simulink model "irep_single_axis"  (Simulink 7.5)
settings: Solver=ode3  StartTime=0.0  StopTime=inf  FixedStep=dt  RelTol=1e-3
InitFcn:
  | IREPOLD_DEPENDENCY
  | init_omni
  | init_filters
  | init_invivo
  | init_telemanipulation
  | init_parker_xyz
  | init_magnetic_tracker
  | init_loadcell
  | init_scopes
  | init_homing
  | init_force_control
  | ATI_Init_nano17
undefined symbols (not defined in the file): A, ATI_torque_convert_to_Nmm, counter_offset, DiscIntNeverNeededParam, dt, encoder_counts, filter_coeffs_ATI, filter_coeffs_ATI_bias, gear_ratio, HomingFineEps, HomingRoughEps, HomingRoughVelocity, inv_T, joystick_filter_coeffs, K_d, K_i, K_p, left_arm_home_voltage, N_ATI, N_ATI_bias, N_joystick, N_pots, pots_filter_coeffs, quadrature_mode, right_arm_home_voltage, RightArmHomingDirectionVector, RightArmHomingIntGain, screw_pitch
libraries: xpcconteclib x23, xpcmeasurementcomputinglib x17, xpclib x11, simulink x8, dspswit3 x4, dspsigops x1, powerlib_extras x1
(part 2 of 3)

== system irep_single_axis/In-Vivo System/CONTEC CARDS/Level 3 ==
  Mux : Mux  Inputs=5
  camera: open joint : xpcconteclib/Incremental Encoder/CNT32-8M(PCI)   Channel=5  OperationMode=2-phase Input Synchronous Clear Multiply by 4  DigitalFilter=No filtering  PulseInput=TTL level input  Direction=Up in the clockwise direction/Down in the counterclockwise direction  InitialValue=counter_offset_init  LoadInitialValue=on  SampleTime=dt  PciSlot=[2,11]  StartMethod=Model Start  StopMethod=Model Terminate  ZeroClearRising=off  ZeroClearFalling=off  ZeroClearMatch0=off  ZeroClearMatch1=off  PresetRising=off  PresetFalling=off  PresetMatch0=off  PresetMatch1=off  PresetValue=0  Match0Value=0  Match1Value=0  OutputSignalMatch0=off  OutputSignalMatch1=off  OutputSignalAbnormal=off  OutputSignalDigitalFilter=off  OutputSignalAlarm=off  OneShotDuration=10 microseconds  IndexEnable=Disable  IndexLogic=Positive (Active High)  EnableDigitalInput=off  EnableDigitalOutput=off  DigitalOutputInitialValue=None  DigitalOutputFinalValue=None
  camera: open joint1 : xpcconteclib/Incremental Encoder/CNT32-8M(PCI)   Channel=6  OperationMode=2-phase Input Synchronous Clear Multiply by 4  DigitalFilter=No filtering  PulseInput=TTL level input  Direction=Up in the clockwise direction/Down in the counterclockwise direction  InitialValue=counter_offset_init  LoadInitialValue=on  SampleTime=dt  PciSlot=[2,11]  StartMethod=Model Start  StopMethod=Model Terminate  ZeroClearRising=off  ZeroClearFalling=off  ZeroClearMatch0=off  ZeroClearMatch1=off  PresetRising=off  PresetFalling=off  PresetMatch0=off  PresetMatch1=off  PresetValue=0  Match0Value=0  Match1Value=0  OutputSignalMatch0=off  OutputSignalMatch1=off  OutputSignalAbnormal=off  OutputSignalDigitalFilter=off  OutputSignalAlarm=off  OneShotDuration=10 microseconds  IndexEnable=Disable  IndexLogic=Positive (Active High)  EnableDigitalInput=off  EnableDigitalOutput=off  DigitalOutputInitialValue=None  DigitalOutputFinalValue=None
  camera: open joint2 : xpcconteclib/Incremental Encoder/CNT32-8M(PCI)   Channel=7  OperationMode=2-phase Input Synchronous Clear Multiply by 4  DigitalFilter=No filtering  PulseInput=TTL level input  Direction=Up in the clockwise direction/Down in the counterclockwise direction  InitialValue=counter_offset_init  LoadInitialValue=on  SampleTime=dt  PciSlot=[2,11]  StartMethod=Model Start  StopMethod=Model Terminate  ZeroClearRising=off  ZeroClearFalling=off  ZeroClearMatch0=off  ZeroClearMatch1=off  PresetRising=off  PresetFalling=off  PresetMatch0=off  PresetMatch1=off  PresetValue=0  Match0Value=0  Match1Value=0  OutputSignalMatch0=off  OutputSignalMatch1=off  OutputSignalAbnormal=off  OutputSignalDigitalFilter=off  OutputSignalAlarm=off  OneShotDuration=10 microseconds  IndexEnable=Disable  IndexLogic=Positive (Active High)  EnableDigitalInput=off  EnableDigitalOutput=off  DigitalOutputInitialValue=None  DigitalOutputFinalValue=None
  left arm: insertion : xpcconteclib/Incremental Encoder/CNT32-8M(PCI)   Channel=4  OperationMode=2-phase Input Synchronous Clear Multiply by 4  DigitalFilter=No filtering  PulseInput=TTL level input  Direction=Up in the clockwise direction/Down in the counterclockwise direction  InitialValue=counter_offset_init  LoadInitialValue=on  SampleTime=dt  PciSlot=[2,11]  StartMethod=Model Start  StopMethod=Model Terminate  ZeroClearRising=off  ZeroClearFalling=off  ZeroClearMatch0=off  ZeroClearMatch1=off  PresetRising=off  PresetFalling=off  PresetMatch0=off  PresetMatch1=off  PresetValue=0  Match0Value=0  Match1Value=0  OutputSignalMatch0=off  OutputSignalMatch1=off  OutputSignalAbnormal=off  OutputSignalDigitalFilter=off  OutputSignalAlarm=off  OneShotDuration=10 microseconds  IndexEnable=Disable  IndexLogic=Positive (Active High)  EnableDigitalInput=off  EnableDigitalOutput=off  DigitalOutputInitialValue=None  DigitalOutputFinalValue=None
  right arm: insertion : xpcconteclib/Incremental Encoder/CNT32-8M(PCI)   Channel=1  OperationMode=2-phase Input Synchronous Clear Multiply by 4  DigitalFilter=No filtering  PulseInput=TTL level input  Direction=Up in the clockwise direction/Down in the counterclockwise direction  InitialValue=counter_offset_init  LoadInitialValue=on  SampleTime=dt  PciSlot=[2,11]  StartMethod=Model Start  StopMethod=Model Terminate  ZeroClearRising=off  ZeroClearFalling=off  ZeroClearMatch0=off  ZeroClearMatch1=off  PresetRising=on  PresetFalling=off  PresetMatch0=off  PresetMatch1=off  PresetValue=0  Match0Value=0  Match1Value=0  OutputSignalMatch0=off  OutputSignalMatch1=off  OutputSignalAbnormal=off  OutputSignalDigitalFilter=off  OutputSignalAlarm=off  OneShotDuration=10 microseconds  IndexEnable=Disable  IndexLogic=Positive (Active High)  EnableDigitalInput=off  EnableDigitalOutput=off  DigitalOutputInitialValue=None  DigitalOutputFinalValue=None
  Out1 : Outport
  wires:
  Mux/1 -> Out1/1
  left arm: insertion/1 -> Mux/2
  right arm: insertion/1 -> Mux/1
  camera: open joint/1 -> Mux/3
  camera: open joint1/1 -> Mux/4
  camera: open joint2/1 -> Mux/5

== system irep_single_axis/In-Vivo System/CONTEC CARDS/RZ ==
  CNT32-8M(PCI) Ch1 : xpcconteclib/Incremental Encoder/CNT32-8M(PCI)   Channel=1  OperationMode=2-phase Input Synchronous Clear Multiply by 4  DigitalFilter=No filtering  PulseInput=Differential line receiver input  Direction=Up in the clockwise direction/Down in the counterclockwise direction  InitialValue=counter_offset  LoadInitialValue=on  SampleTime=dt  PciSlot=[2 14]  StartMethod=Model Start  StopMethod=Model Terminate  ZeroClearRising=off  ZeroClearFalling=off  ZeroClearMatch0=off  ZeroClearMatch1=off  PresetRising=off  PresetFalling=off  PresetMatch0=off  PresetMatch1=off  PresetValue=0  Match0Value=0  Match1Value=0  OutputSignalMatch0=off  OutputSignalMatch1=off  OutputSignalAbnormal=off  OutputSignalDigitalFilter=off  OutputSignalAlarm=off  OneShotDuration=10 microseconds  IndexEnable=Disable  IndexLogic=Positive (Active High)  EnableDigitalInput=off  EnableDigitalOutput=off  DigitalOutputInitialValue=None  DigitalOutputFinalValue=None
  CNT32-8M(PCI) Ch2 : xpcconteclib/Incremental Encoder/CNT32-8M(PCI)   Channel=2  OperationMode=2-phase Input Synchronous Clear Multiply by 4  DigitalFilter=No filtering  PulseInput=Differential line receiver input  Direction=Up in the clockwise direction/Down in the counterclockwise direction  InitialValue=counter_offset  LoadInitialValue=on  SampleTime=dt  PciSlot=[2 14]  StartMethod=Model Start  StopMethod=Model Terminate  ZeroClearRising=off  ZeroClearFalling=off  ZeroClearMatch0=off  ZeroClearMatch1=off  PresetRising=off  PresetFalling=off  PresetMatch0=off  PresetMatch1=off  PresetValue=0  Match0Value=0  Match1Value=0  OutputSignalMatch0=off  OutputSignalMatch1=off  OutputSignalAbnormal=off  OutputSignalDigitalFilter=off  OutputSignalAlarm=off  OneShotDuration=10 microseconds  IndexEnable=Disable  IndexLogic=Positive (Active High)  EnableDigitalInput=off  EnableDigitalOutput=off  DigitalOutputInitialValue=None  DigitalOutputFinalValue=None
  Mux : Mux  Inputs=2
  Out1 : Outport
  wires:
  CNT32-8M(PCI) Ch2/1 -> Mux/2
  CNT32-8M(PCI) Ch1/1 -> Mux/1
  Mux/1 -> Out1/1

== system irep_single_axis/In-Vivo System/Count to mm/Bus Creator ==
  In1 : Inport
  Bus Creator : BusCreator  Inputs=23
  Demux : Demux  Outputs=23
  Out1 : Outport
  wires:
  Demux/1 -> Bus Creator/1  "Righ arm - Proximal segment - bending in Y"
  Demux/2 -> Bus Creator/2  "Right arm - Gripper Joint"
  Demux/3 -> Bus Creator/3  "Right arm - Proximal segment - bending in X"
  Demux/4 -> Bus Creator/4  "Right arm - distal segment - bending in X"
  Demux/5 -> Bus Creator/5  "Right arm - wrist"
  Demux/6 -> Bus Creator/6  "Right arm - distal segment - bending in Y"
  Demux/7 -> Bus Creator/7  "Right arm - parallelogram deployment joint"
  Demux/8 -> Bus Creator/8  "Right arm - parallelogram insert joint"
  Demux/9 -> Bus Creator/9  "Left arm - proximal segment - bending in Y"
  Demux/10 -> Bus Creator/10  "Left arm - gripper joint"
  Demux/11 -> Bus Creator/11  "Left arm - proximal segment - bending in X"
  Demux/12 -> Bus Creator/12  "Left arm - distal segment - bending in x"
  Demux/13 -> Bus Creator/13  "Left arm - wrist"
  Demux/14 -> Bus Creator/14  "Left arm - distal segment - bending in y"
  Demux/15 -> Bus Creator/15  "Left arm - parallelogram deployment joint"
  Demux/16 -> Bus Creator/16  "Left arm - parallelogram insert joint"
  Demux/17 -> Bus Creator/17  "Right arm - overall translational movement"
  Demux/18 -> Bus Creator/18  "Left arm - overall translational movement"
  Demux/19 -> Bus Creator/19  "Camera shell open"
  Demux/20 -> Bus Creator/20  "Camera Pan"
  Demux/21 -> Bus Creator/21  "Camera Tilt"
  Bus Creator/1 -> Out1/1
  In1/1 -> Demux/1
  Demux/22 -> Bus Creator/22  "Parker insertion stage"
  Demux/23 -> Bus Creator/23  "Parker rotary stage"

== system irep_single_axis/In-Vivo System/D/A/Bus Selector 1 ==
  In1 : Inport
  Bus Selector : BusSelector  OutputSignals=Right arm - Proximal Segment Y,Right arm - Gripper Joint,Right arm - Proximal Segment X,Right arm - Distal Segment X,Right arm - Wrist Joint,Right arm - Distal Segment Y,Right arm - Parallelogram Deploy,Right arm - Parallelogram Insert
  Gain{,1..3} (4 alike) : Gain  Gain=-1  ParameterDataType=fixdt(1, 16)  ParameterScaling=2^0  OutDataType=fixdt(1, 16)  OutScaling=2^0
  Mux : Mux  Inputs=8
  Out1 : Outport
  wires:
  Bus Selector/1 -> Mux/1  "<Right arm - Proximal Segment Y>"
  Bus Selector/2 -> Mux/2  "<Right arm - Gripper Joint>"
  Bus Selector/3 -> Gain/1  "<Right arm - Proximal Segment X>"
  Bus Selector/4 -> Gain1/1  "<Right arm - Distal Segment X>"
  Bus Selector/5 -> Mux/5  "<Right arm - Wrist Joint>"
  Bus Selector/6 -> Mux/6  "<Right arm - Distal Segment Y>"
  Bus Selector/7 -> Gain2/1  "<Right arm - Parallelogram Deploy>"
  Bus Selector/8 -> Gain3/1  "<Right arm - Parallelogram Insert>"
  In1/1 -> Bus Selector/1
  Mux/1 -> Out1/1
  Gain/1 -> Mux/3
  Gain1/1 -> Mux/4
  Gain2/1 -> Mux/7
  Gain3/1 -> Mux/8

== system irep_single_axis/In-Vivo System/D/A/Bus Selector 2 ==
  In1 : Inport
  Bus Selector : BusSelector  OutputSignals=Left arm - Proximal Segment Y,Left arm - Gripper Joint,Left arm - Proximal Segment X,Left arm - Distal Segment X,Left arm - Wrist Joint,Left arm - Distal Segment Y,Left arm - Parallelogram Deploy,Left arm - Parallelogram Insert
  Gain{1..4} (4 alike) : Gain  Gain=-1  ParameterDataType=fixdt(1, 16)  ParameterScaling=2^0  OutDataType=fixdt(1, 16)  OutScaling=2^0
  Mux : Mux  Inputs=8
  Out1 : Outport
  wires:
  Bus Selector/1 -> Gain1/1  "<Left arm - Proximal Segment Y>"
  Bus Selector/2 -> Mux/2  "<Left arm - Gripper Joint>"
  Bus Selector/4 -> Mux/4  "<Left arm - Distal Segment X>"
  Bus Selector/5 -> Mux/5  "<Left arm - Wrist Joint>"
  Bus Selector/6 -> Gain2/1  "<Left arm - Distal Segment Y>"
  Bus Selector/7 -> Gain3/1  "<Left arm - Parallelogram Deploy>"
  Bus Selector/8 -> Gain4/1  "<Left arm - Parallelogram Insert>"
  In1/1 -> Bus Selector/1
  Mux/1 -> Out1/1
  Bus Selector/3 -> Mux/3  "<Left arm - Proximal Segment X>"
  Gain1/1 -> Mux/1
  Gain2/1 -> Mux/6
  Gain3/1 -> Mux/7
  Gain4/1 -> Mux/8

== system irep_single_axis/In-Vivo System/D/A/Bus Selector 3 ==
  In1 : Inport
  Bus Selector : BusSelector  OutputSignals=Righ arm - Overall Translational Movement,Left arm - Overall Translational Movement,Camera shell open,Camera Pan,Camera Tilt
  Mux : Mux  Inputs=5
  Out1 : Outport
  wires:
  Mux/1 -> Out1/1
  In1/1 -> Bus Selector/1
  Bus Selector/1 -> Mux/1  "<Righ arm - Overall Translational Movement>"
  Bus Selector/2 -> Mux/2  "<Left arm - Overall Translational Movement>"
  Bus Selector/3 -> Mux/3  "<Camera shell open>"
  Bus Selector/4 -> Mux/4  "<Camera Pan>"
  Bus Selector/5 -> Mux/5  "<Camera Tilt>"

== system irep_single_axis/In-Vivo System/D/A/Level 1 ==
  In1 : Inport
  Demux1 : Demux  Outputs=8
  Level 1 : xpcmeasurementcomputinglib/D//A/PCI-DDA08 12   channel=[1,2,3,4,5,6,7,8]  range=[-10,-10,-10,-10,-10,-10,-10,-10]  reset=[1,1,1,1,1,1,1,1]  initValue=[0,0,0,0,0,0,0,0]  sampletime=dt  pci_dev=[2, 7]
  wires:
  Demux1/1 -> Level 1/1
  Demux1/2 -> Level 1/2
  Demux1/3 -> Level 1/3
  Demux1/4 -> Level 1/4
  Demux1/5 -> Level 1/5
  Demux1/6 -> Level 1/6
  Demux1/7 -> Level 1/7
  Demux1/8 -> Level 1/8
  In1/1 -> Demux1/1

== system irep_single_axis/In-Vivo System/D/A/Level 2 ==
  In1 : Inport
  Demux2 : Demux  Outputs=8
  Level 2 : xpcmeasurementcomputinglib/D//A/PCI-DDA08 12   channel=[1,2,3,4,5,6,7,8]  range=[-10,-10,-10,-10,-10,-10,-10,-10]  reset=[1,1,1,1,1,1,1,1]  initValue=[0,0,0,0,0,0,0,0]  sampletime=dt  pci_dev=[2, 10]
  wires:
  Demux2/1 -> Level 2/1
  Demux2/2 -> Level 2/2
  Demux2/3 -> Level 2/3
  Demux2/4 -> Level 2/4
  Demux2/5 -> Level 2/5
  Demux2/6 -> Level 2/6
  Demux2/7 -> Level 2/7
  Demux2/8 -> Level 2/8
  In1/1 -> Demux2/1

== system irep_single_axis/In-Vivo System/D/A/Level 3 ==
  In1 : Inport
  Demux1 : Demux  Outputs=5
  Level 3 : xpcmeasurementcomputinglib/D//A/PCI-DDA08 12   channel=[1,2,3,4,5,6,7]  range=[-10,-10,-10,-10,-10,-10,-10]  reset=[1,1,1,1,1,1,1]  initValue=[0,0,0,0,0,0,0]  sampletime=dt  pci_dev=[2, 13]
  wires:
  In1/1 -> Demux1/1
  Demux1/1 -> Level 3/1
  Demux1/2 -> Level 3/4
  Demux1/3 -> Level 3/5
  Demux1/4 -> Level 3/6
  Demux1/5 -> Level 3/7

== system irep_single_axis/In-Vivo System/Potentiometers/Filter ==
  in : Inport  OutDataType=sfix(16)  OutScaling=2^0
  Discrete FIR Filter : DiscreteFir  CoefSource=Input port
  Gain : Gain  Gain=1/N_pots  ParameterDataType=sfix(16)  ParameterScaling=2^0  OutDataType=sfix(16)  OutScaling=2^0
  vel_filter_coeffs : Constant  Value=pots_filter_coeffs  OutDataType=sfix(16)  OutScaling=2^0
  out : Outport  OutDataType=sfix(16)  OutScaling=2^0
  wires:
  in/1 -> Discrete FIR Filter/1
  Gain/1 -> out/1
  vel_filter_coeffs/1 -> Discrete FIR Filter/2
  Discrete FIR Filter/1 -> Gain/1

== system irep_single_axis/In-Vivo System/Potentiometers/Filter1 ==
  in : Inport  OutDataType=sfix(16)  OutScaling=2^0
  Discrete FIR Filter : DiscreteFir  CoefSource=Input port
  Gain : Gain  Gain=1/N_pots  ParameterDataType=sfix(16)  ParameterScaling=2^0  OutDataType=sfix(16)  OutScaling=2^0
  vel_filter_coeffs : Constant  Value=pots_filter_coeffs  OutDataType=sfix(16)  OutScaling=2^0
  out : Outport  OutDataType=sfix(16)  OutScaling=2^0
  wires:
  Discrete FIR Filter/1 -> Gain/1
  vel_filter_coeffs/1 -> Discrete FIR Filter/2
  Gain/1 -> out/1
  in/1 -> Discrete FIR Filter/1

== system irep_single_axis/In-Vivo System/Potentiometers/Filter2 ==
  in : Inport  OutDataType=sfix(16)  OutScaling=2^0
  Discrete FIR Filter : DiscreteFir  CoefSource=Input port
  Gain : Gain  Gain=1/N_pots  ParameterDataType=sfix(16)  ParameterScaling=2^0  OutDataType=sfix(16)  OutScaling=2^0
  vel_filter_coeffs : Constant  Value=pots_filter_coeffs  OutDataType=sfix(16)  OutScaling=2^0
  out : Outport  OutDataType=sfix(16)  OutScaling=2^0
  wires:
  Discrete FIR Filter/1 -> Gain/1
  vel_filter_coeffs/1 -> Discrete FIR Filter/2
  Gain/1 -> out/1
  in/1 -> Discrete FIR Filter/1

== system irep_single_axis/In-Vivo System/Potentiometers/Filter3 ==
  in : Inport  OutDataType=sfix(16)  OutScaling=2^0
  Discrete FIR Filter : DiscreteFir  CoefSource=Input port
  Gain : Gain  Gain=1/N_joystick  ParameterDataType=sfix(16)  ParameterScaling=2^0  OutDataType=sfix(16)  OutScaling=2^0
  vel_filter_coeffs : Constant  Value=joystick_filter_coeffs  OutDataType=sfix(16)  OutScaling=2^0
  out : Outport  OutDataType=sfix(16)  OutScaling=2^0
  wires:
  in/1 -> Discrete FIR Filter/1
  Gain/1 -> out/1
  vel_filter_coeffs/1 -> Discrete FIR Filter/2
  Discrete FIR Filter/1 -> Gain/1

== system irep_single_axis/In-Vivo System/Potentiometers/Initialize Joystick ==
  In1 : Inport
  Digital Clock : DigitalClock  SampleTime=dt
  Embedded MATLAB Function : Stateflow chart  TreatAsAtomicUnit=on
  Unit Delay : UnitDelay  X0=zeros(3,1)  SampleTime=dt
  Out1 : Outport
  wires:
  Digital Clock/1 -> Embedded MATLAB Function/2(t)
  Unit Delay/1 -> Embedded MATLAB Function/3(u_prev)
  In1/1 -> Embedded MATLAB Function/1(u_curr)
  Embedded MATLAB Function/1(V) -> Out1/1  "camer"
  Embedded MATLAB Function/2(v_zero) -> Unit Delay/1  "camera joystick"

== system irep_single_axis/Joint Level PID Control in mm/Bus selector/Camera selector ==
  In1 : Inport
  Bus Selector : BusSelector  OutputSignals=q.Camera shell open,q.Camera Pan,q.Camera Tilt
  Mux : Mux  Inputs=3
  Out1 : Outport
  wires:
  Mux/1 -> Out1/1
  In1/1 -> Bus Selector/1
  Bus Selector/3 -> Mux/3  "<Camera Tilt>"
  Bus Selector/2 -> Mux/2  "<Camera Pan>"
  Bus Selector/1 -> Mux/1  "<Camera shell open>"

== system irep_single_axis/Joint Level PID Control in mm/Bus selector/Left arm selector ==
  In1 : Inport
  Bus Selector : BusSelector  OutputSignals=q.Left arm - overall translational movement,q.Left arm - parallelogram insert joint,q.Left arm - parallelogram deployment joint,q.Left arm - proximal segment - bending in X,q.Left arm - proximal segment - bending in Y,q.Left arm - distal segment - bending in x,q.Left arm - distal segment - bending in y,q.Left arm - wrist,q.Left arm - gripper joint
  Mux : Mux  Inputs=9
  Out1 : Outport
  wires:
  In1/1 -> Bus Selector/1
  Mux/1 -> Out1/1
  Bus Selector/1 -> Mux/1  "<Left arm - overall translational movement>"
  Bus Selector/2 -> Mux/2  "<Left arm - parallelogram insert joint>"
  Bus Selector/3 -> Mux/3  "<Left arm - parallelogram deployment joint>"
  Bus Selector/4 -> Mux/4  "<Left arm - proximal segment - bending in X>"
  Bus Selector/5 -> Mux/5  "<Left arm - proximal segment - bending in Y>"
  Bus Selector/8 -> Mux/8  "<Left arm - wrist>"
  Bus Selector/9 -> Mux/9  "<Left arm - gripper joint>"
  Bus Selector/6 -> Mux/6  "<Left arm - distal segment - bending in x>"
  Bus Selector/7 -> Mux/7  "<Left arm - distal segment - bending in y>"

== system irep_single_axis/Joint Level PID Control in mm/Bus selector/RZ ==
  In1 : Inport
  Bus Selector : BusSelector  OutputSignals=q.Parker insertion stage,q.Parker rotary stage
  Mux : Mux  Inputs=2
  Out1 : Outport
  wires:
  Mux/1 -> Out1/1
  In1/1 -> Bus Selector/1
  Bus Selector/2 -> Mux/2  "<Parker rotary stage>"
  Bus Selector/1 -> Mux/1  "<Parker insertion stage>"

== system irep_single_axis/Joint Level PID Control in mm/Bus selector/Right arm  selector ==
  In1 : Inport
  Bus Selector : BusSelector  OutputSignals=q.Right arm - overall translational movement,q.Right arm - parallelogram insert joint,q.Right arm - parallelogram deployment joint,q.Right arm - Proximal segment - bending in X,q.Righ arm - Proximal segment - bending in Y,q.Right arm - distal segment - bending in X,q.Right arm - distal segment - bending in Y,q.Right arm - wrist,q.Right arm - Gripper Joint
  Mux : Mux  Inputs=9
  Out1 : Outport
  wires:
  In1/1 -> Bus Selector/1
  Mux/1 -> Out1/1
  Bus Selector/1 -> Mux/1  "<Right arm - overall translational movement>"
  Bus Selector/2 -> Mux/2  "<Right arm - parallelogram insert joint>"
  Bus Selector/3 -> Mux/3  "<Right arm - parallelogram deployment joint>"
  Bus Selector/4 -> Mux/4  "<Right arm - Proximal segment - bending in X>"
  Bus Selector/5 -> Mux/5  "<Righ arm - Proximal segment - bending in Y>"
  Bus Selector/6 -> Mux/6  "<Right arm - distal segment - bending in X>"
  Bus Selector/7 -> Mux/7  "<Right arm - distal segment - bending in Y>"
  Bus Selector/8 -> Mux/8  "<Right arm - wrist>"
  Bus Selector/9 -> Mux/9  "<Right arm - Gripper Joint>"

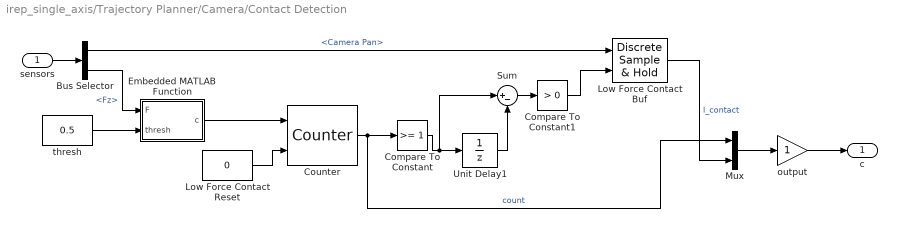
== system irep_single_axis/Trajectory Planner/Camera/Contact Detection ==
  sensors : Inport  OutDataType=fixdt(1, 16)  OutScaling=2^0
  Bus Selector : BusSelector  OutputSignals=q.Camera Pan,ATI.Fz
  Compare To Constant : simulink/Logic and Bit Operations/Compare To Constant  SystemSampleTime=-1  relop=>=  const=1  LogicOutDataTypeMode=boolean
  Compare To Constant1 : simulink/Logic and Bit Operations/Compare To Constant  SystemSampleTime=-1  relop=>  const=0  LogicOutDataTypeMode=boolean
  Counter : dspswit3/Counter  Direction=Up  CountEvent=Rising edge  CounterSize=32 bits  MaxCount=255  InitialCount=0  Output=Count  HitValue=32  ResetInput=on  SamplesPerFrame=1  Ts=1  CntDtype=double  HitDtype=Logical
  Embedded MATLAB Function : Stateflow chart  TreatAsAtomicUnit=on
  Low Force Contact Buf : powerlib_extras/Discrete  Control Blocks/Discrete Sample & Hold  DialogController=POWERSYS.PowerSysDialog  SystemSampleTime=-1  ic=0  Ts=dt
  Low Force Contact Reset : Constant  Value=0
  Mux : Mux  Inputs=2
  Sum : Sum  Inputs=|+-
  Unit Delay1 : UnitDelay  SampleTime=-1
  output : Gain  ParameterDataType=fixdt(1, 16)  ParameterScaling=2^0  OutDataType=fixdt(1, 16)  OutScaling=2^0
  thresh : Constant  Value=0.5
  c : Outport  OutDataType=fixdt(1, 16)  OutScaling=2^0
  wires:
  Embedded MATLAB Function/1(c) -> Counter/1
  Low Force Contact Buf/1 -> Mux/2  "l_contact"
  Low Force Contact Reset/1 -> Counter/2
  Counter/1 -> Mux/1, Compare To Constant/1  "count"
  Unit Delay1/1 -> Sum/2
  Compare To Constant/1 -> Sum/1, Unit Delay1/1
  Sum/1 -> Compare To Constant1/1
  Compare To Constant1/1 -> Low Force Contact Buf/2
  Mux/1 -> output/1
  sensors/1 -> Bus Selector/1
  Bus Selector/1 -> Low Force Contact Buf/1  "<Camera Pan>"
  Bus Selector/2 -> Embedded MATLAB Function/1(F)  "<Fz>"
  thresh/1 -> Embedded MATLAB Function/2(thresh)
  output/1 -> c/1

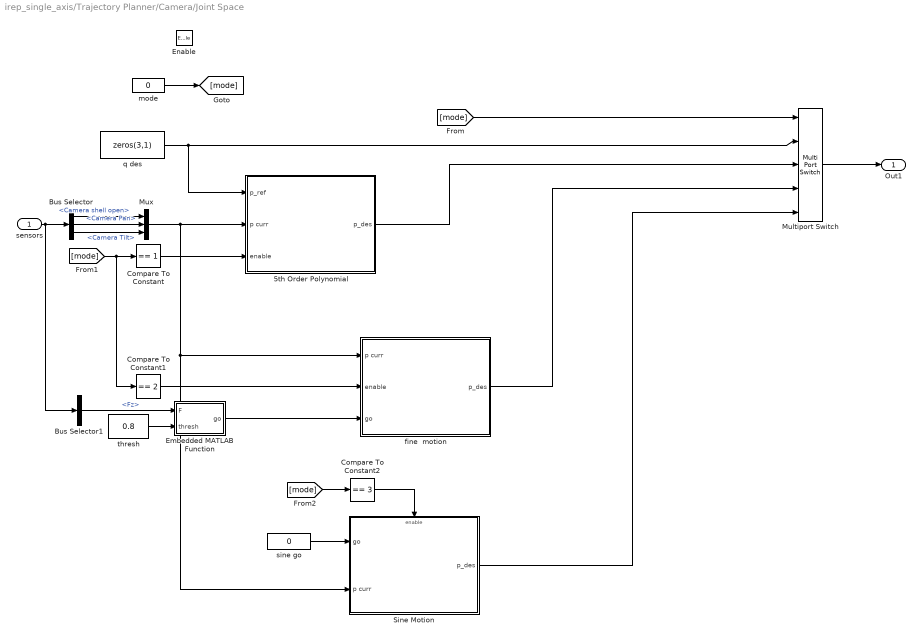
== system irep_single_axis/Trajectory Planner/Camera/Joint Space ==
  sensors : Inport  OutDataType=fixdt(1, 16)  OutScaling=2^0
  Enable : EnablePort
  5th Order Polynomial : Subsystem
  Bus Selector : BusSelector  OutputSignals=q.Camera shell open,q.Camera Pan,q.Camera Tilt
  Bus Selector1 : BusSelector  OutputSignals=ATI.Fz
  Compare To Constant : simulink/Logic and Bit Operations/Compare To Constant  SystemSampleTime=-1  relop===  const=1  LogicOutDataTypeMode=uint8
  Compare To Constant1 : simulink/Logic and Bit Operations/Compare To Constant  SystemSampleTime=-1  relop===  const=2  LogicOutDataTypeMode=uint8
  Compare To Constant2 : simulink/Logic and Bit Operations/Compare To Constant  SystemSampleTime=-1  relop===  const=3  LogicOutDataTypeMode=uint8
  Embedded MATLAB Function : Stateflow chart  TreatAsAtomicUnit=on
  Multiport Switch : MultiPortSwitch  DataPortOrder=Zero-based contiguous  Inputs=4  zeroidx=on  OutDataType=fixdt(1, 16)  OutScaling=2^0
  Mux : Mux  Inputs=3
  Sine Motion : Subsystem
  fine  motion : Subsystem
  mode : Constant  Value=0  OutDataType=fixdt(1, 16)  OutScaling=2^0  SampleTime=dt
  q des : Constant  Value=zeros(3,1)  OutDataType=fixdt(1, 16)  OutScaling=2^0  SampleTime=dt
  sine go : Constant  Value=0  OutDataType=fixdt(1, 16)  OutScaling=2^0  SampleTime=dt
  thresh : Constant  Value=0.8
  Out1 : Outport  OutDataType=fixdt(1, 16)  OutScaling=2^0
  wires:
  q des/1 -> 5th Order Polynomial/1(p_ref), Multiport Switch/2
  sensors/1 -> Bus Selector/1, Bus Selector1/1
  Bus Selector/1 -> Mux/1  "<Camera shell open>"
  Bus Selector/2 -> Mux/2  "<Camera Pan>"
  Bus Selector/3 -> Mux/3  "<Camera Tilt>"
  Mux/1 -> 5th Order Polynomial/2(p curr), fine  motion/1(p curr), Sine Motion/2(p curr)
  Multiport Switch/1 -> Out1/1
  5th Order Polynomial/1(p_des) -> Multiport Switch/3
  mode/1 -> [mode]
  [mode] -> Multiport Switch/1
  [mode] -> Compare To Constant/1, Compare To Constant1/1
  Compare To Constant/1 -> 5th Order Polynomial/3(enable)
  fine  motion/1(p_des) -> Multiport Switch/4
  Compare To Constant1/1 -> fine  motion/2(enable)
  Bus Selector1/1 -> Embedded MATLAB Function/1(F)  "<Fz>"
  thresh/1 -> Embedded MATLAB Function/2(thresh)
  Embedded MATLAB Function/1(go) -> fine  motion/3(go)
  [mode] -> Compare To Constant2/1
  Compare To Constant2/1 -> Sine Motion/Enable
  sine go/1 -> Sine Motion/1(go)
  Sine Motion/1(p_des) -> Multiport Switch/5

== system irep_single_axis/Trajectory Planner/Left Arm/Low Level ==
  sensors : Inport  OutDataType=fixdt(1, 16)  OutScaling=2^0
  Enable : EnablePort
  Bus Selector : BusSelector  OutputSignals=Pots_Connect.L_Pots_Connect
  Enable Home Procedure : Constant  Value=0  OutDataType=fixdt(1, 16)  OutScaling=2^0  SampleTime=dt
  Enable Joint Space : Constant  Value=0  OutDataType=fixdt(1, 16)  OutScaling=2^0  SampleTime=dt
  Home Procedure : Subsystem  TreatAsAtomicUnit=on
  Home Procedure2 : Subsystem  TreatAsAtomicUnit=on
  Joint Space : Subsystem  TreatAsAtomicUnit=on
  Merge1 : Merge  InitialOutput=zeros(9,1)
  Not And : Stateflow chart  TreatAsAtomicUnit=on
  q des : Outport  OutDataType=fixdt(1, 16)  OutScaling=2^0
  wires:
  sensors/1 -> Bus Selector/1, Home Procedure2/1(sensors), Home Procedure/1(sensors)
  Merge1/1 -> q des/1
  Enable Joint Space/1 -> Joint Space/Enable
  Joint Space/1(q des) -> Merge1/2
  Bus Selector/1 -> Not And/1(connected)  "<L_Pots_Connect>"
  Enable Home Procedure/1 -> Not And/2(enable_home)
  Not And/1(enable) -> Home Procedure2/Enable, Home Procedure/Enable
  Home Procedure/1(q des) -> Merge1/1

== system irep_single_axis/Trajectory Planner/Right Arm/Low Level ==
  sensors : Inport  OutDataType=fixdt(1, 16)  OutScaling=2^0
  Enable : EnablePort
  Bus Selector : BusSelector  OutputSignals=Pots_Connect.R_Pots_Connect
  Enable Home Procedure : Constant  Value=0  OutDataType=fixdt(1, 16)  OutScaling=2^0  SampleTime=dt
  Enable Joint Space : Constant  Value=0  OutDataType=fixdt(1, 16)  OutScaling=2^0  SampleTime=dt
  Home Procedure : Subsystem  TreatAsAtomicUnit=on
  Joint Space : Subsystem  TreatAsAtomicUnit=on
  Merge1 : Merge  InitialOutput=zeros(9,1)
  Not And : Stateflow chart  TreatAsAtomicUnit=on
  q des : Outport  OutDataType=fixdt(1, 16)  OutScaling=2^0
  wires:
  sensors/1 -> Home Procedure/1(sensors), Bus Selector/1
  Home Procedure/1(q des) -> Merge1/1
  Enable Joint Space/1 -> Joint Space/Enable
  Joint Space/1(q des) -> Merge1/2
  Merge1/1 -> q des/1
  Bus Selector/1 -> Not And/1(connected)  "<R_Pots_Connect>"
  Not And/1(enable) -> Home Procedure/Enable
  Enable Home Procedure/1 -> Not And/2(enable_home)

== system irep_single_axis/In-Vivo System/ATI FT Sensor/ATI Force Torque Sensor/Enabled Subsystem ==
  In1 : Inport
  Enable : EnablePort
  Data Store Write : DataStoreWrite  DataStoreName=A  SampleTime=-1
  wires:
  In1/1 -> Data Store Write/1

== system irep_single_axis/In-Vivo System/ATI FT Sensor/ATI Force Torque Sensor/Enabled Subsystem1 ==
  In1 : Inport
  Enable : EnablePort
  Voltage Filter Bias : Subsystem
  Out1 : Outport
  wires:
  In1/1 -> Voltage Filter Bias/1(V_in)
  Voltage Filter Bias/1(V_Out) -> Out1/1

== system irep_single_axis/In-Vivo System/ATI FT Sensor/ATI Force Torque Sensor/Voltage Filter ==
  V_in : Inport
  Discrete FIR Filter : DiscreteFir  CoefSource=Input port
  Gain : Gain  Gain=1/N_ATI
  filter_coeffs : Constant  Value=filter_coeffs_ATI
  V_Out : Outport
  wires:
  V_in/1 -> Discrete FIR Filter/1
  Discrete FIR Filter/1 -> Gain/1
  filter_coeffs/1 -> Discrete FIR Filter/2
  Gain/1 -> V_Out/1

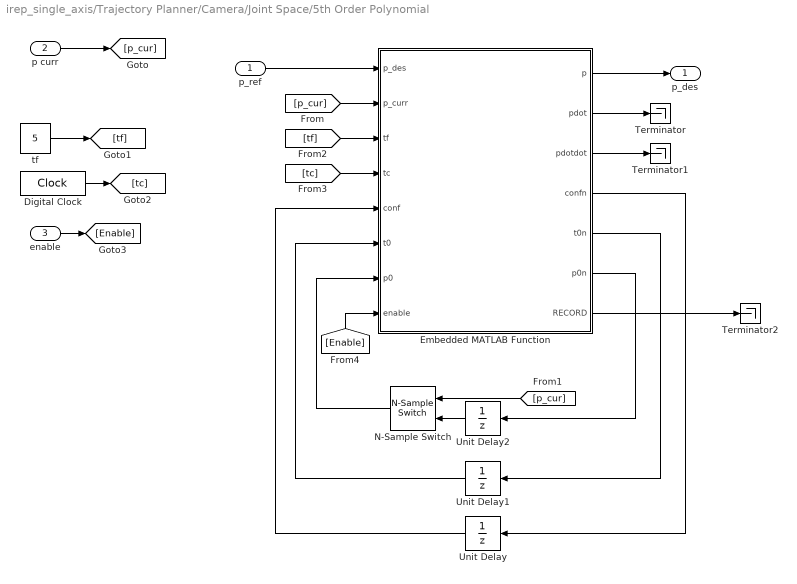
== system irep_single_axis/Trajectory Planner/Camera/Joint Space/5th Order Polynomial ==
  p_ref : Inport
  p curr : Inport  Port=2
  enable : Inport  Port=3
  Digital Clock : DigitalClock  SampleTime=dt
  Embedded MATLAB Function : Stateflow chart  TreatAsAtomicUnit=on
  N-Sample Switch : dspswit3/N-Sample Switch  SystemSampleTime=-1  N=1  reset=off  TriggerType=Rising edge  Ts=dt
  Terminator : Terminator
  Terminator1 : Terminator
  Terminator2 : Terminator
  Unit Delay : UnitDelay  SampleTime=dt
  Unit Delay1 : UnitDelay  SampleTime=dt
  Unit Delay2 : UnitDelay  SampleTime=dt
  tf : Constant  Value=5  SampleTime=dt
  p_des : Outport
  wires:
  Embedded MATLAB Function/4(confn) -> Unit Delay/1
  Unit Delay/1 -> Embedded MATLAB Function/5(conf)
  Embedded MATLAB Function/5(t0n) -> Unit Delay1/1
  Embedded MATLAB Function/6(p0n) -> Unit Delay2/1
  Unit Delay1/1 -> Embedded MATLAB Function/6(t0)
  p_ref/1 -> Embedded MATLAB Function/1(p_des)
  Embedded MATLAB Function/2(pdot) -> Terminator/1
  Embedded MATLAB Function/3(pdotdot) -> Terminator1/1
  N-Sample Switch/1 -> Embedded MATLAB Function/7(p0)
  Unit Delay2/1 -> N-Sample Switch/2
  p curr/1 -> [p_cur]
  [p_cur] -> Embedded MATLAB Function/2(p_curr)
  [p_cur] -> N-Sample Switch/1
  Embedded MATLAB Function/7(RECORD) -> Terminator2/1
  Embedded MATLAB Function/1(p) -> p_des/1
  tf/1 -> [tf]
  Digital Clock/1 -> [tc]
  [tf] -> Embedded MATLAB Function/3(tf)
  [tc] -> Embedded MATLAB Function/4(tc)
  enable/1 -> [Enable]
  [Enable] -> Embedded MATLAB Function/8(enable)

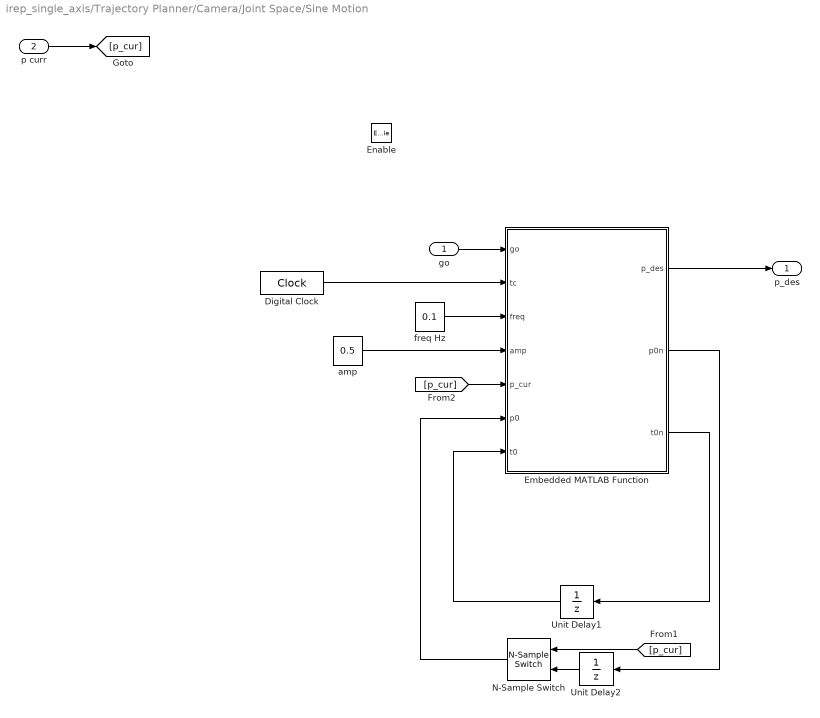
== system irep_single_axis/Trajectory Planner/Camera/Joint Space/Sine Motion ==
  go : Inport
  p curr : Inport  Port=2
  Enable : EnablePort  StatesWhenEnabling=reset
  Digital Clock : DigitalClock  SampleTime=dt
  Embedded MATLAB Function : Stateflow chart  TreatAsAtomicUnit=on
  N-Sample Switch : dspswit3/N-Sample Switch  SystemSampleTime=-1  N=1  reset=off  TriggerType=Rising edge  Ts=dt
  Unit Delay1 : UnitDelay  SampleTime=dt
  Unit Delay2 : UnitDelay  SampleTime=dt
  amp : Constant  Value=0.5  SampleTime=dt
  freq Hz : Constant  Value=0.1  SampleTime=dt
  p_des : Outport
  wires:
  p curr/1 -> [p_cur]
  N-Sample Switch/1 -> Embedded MATLAB Function/6(p0)
  Unit Delay2/1 -> N-Sample Switch/2
  [p_cur] -> N-Sample Switch/1
  Digital Clock/1 -> Embedded MATLAB Function/2(tc)
  freq Hz/1 -> Embedded MATLAB Function/3(freq)
  Embedded MATLAB Function/3(t0n) -> Unit Delay1/1
  Unit Delay1/1 -> Embedded MATLAB Function/7(t0)
  amp/1 -> Embedded MATLAB Function/4(amp)
  Embedded MATLAB Function/2(p0n) -> Unit Delay2/1
  Embedded MATLAB Function/1(p_des) -> p_des/1
  [p_cur] -> Embedded MATLAB Function/5(p_cur)
  go/1 -> Embedded MATLAB Function/1(go)

== system irep_single_axis/Trajectory Planner/Camera/Joint Space/fine  motion ==
  p curr : Inport
  enable : Inport  Port=2
  go : Inport  Port=3
  Embedded MATLAB Function : Stateflow chart  TreatAsAtomicUnit=on
  N-Sample Switch : dspswit3/N-Sample Switch  SystemSampleTime=-1  N=1  reset=off  TriggerType=Rising edge  Ts=dt
  Unit Delay2 : UnitDelay  SampleTime=dt
  dt : Constant  Value=dt  OutDataType=fixdt(1, 16)  OutScaling=2^0  SampleTime=dt
  dt1 : Constant  Value=[0.05;0.05;0.05]  OutDataType=fixdt(1, 16)  OutScaling=2^0  SampleTime=dt
  p_des : Outport
  wires:
  Embedded MATLAB Function/1(p_des) -> p_des/1, Unit Delay2/1
  N-Sample Switch/1 -> Embedded MATLAB Function/6(p_cur)
  enable/1 -> Embedded MATLAB Function/1(enable)
  Unit Delay2/1 -> N-Sample Switch/2
  [p_cur] -> N-Sample Switch/1
  p curr/1 -> [p_cur]
  [p_cur] -> Embedded MATLAB Function/5(p0)
  go/1 -> Embedded MATLAB Function/2(go)
  dt/1 -> Embedded MATLAB Function/3(dt)
  dt1/1 -> Embedded MATLAB Function/4(velocity)

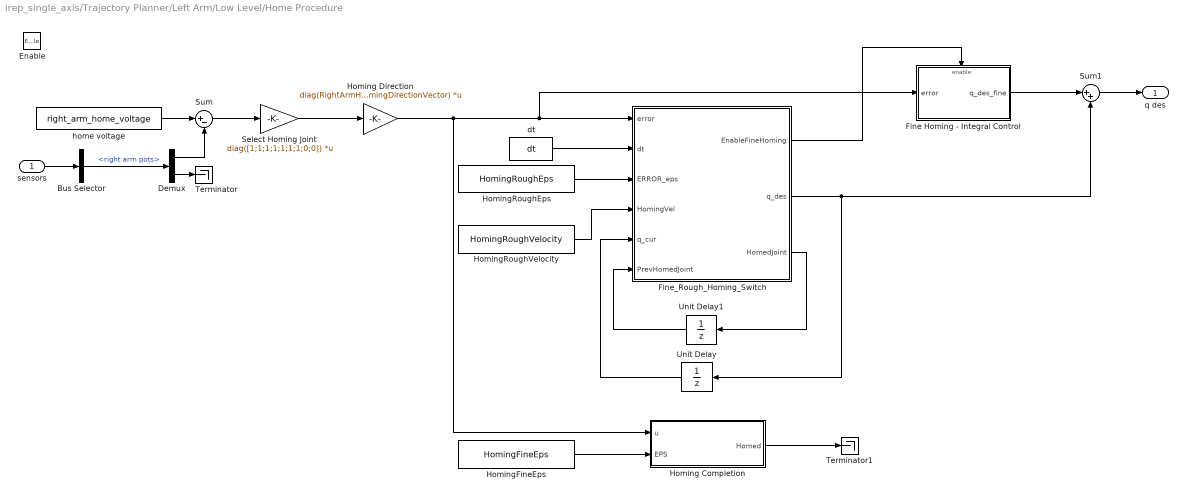
== system irep_single_axis/Trajectory Planner/Left Arm/Low Level/Home Procedure ==
  sensors : Inport  OutDataType=fixdt(1, 16)  OutScaling=2^0
  Enable : EnablePort
  Bus Selector : BusSelector  OutputSignals=A/D signals.right arm pots
  Demux : Demux  Outputs=[9 1]
  Fine Homing - Integral Control : Subsystem
  Fine_Rough_Homing_Switch : Stateflow chart  TreatAsAtomicUnit=on
  Homing Completion : Stateflow chart  TreatAsAtomicUnit=on
  Homing Direction : Gain  Gain=diag(RightArmHomingDirectionVector)  Multiplication=Matrix(K*u)  ParameterDataType=fixdt(1, 16)  ParameterScaling=2^0  OutDataType=fixdt(1, 16)  OutScaling=2^0  SampleTime=dt
  HomingFineEps : Constant  Value=HomingFineEps  OutDataType=fixdt(1, 16)  OutScaling=2^0  SampleTime=dt
  HomingRoughEps : Constant  Value=HomingRoughEps  OutDataType=fixdt(1, 16)  OutScaling=2^0  SampleTime=dt
  HomingRoughVelocity : Constant  Value=HomingRoughVelocity  OutDataType=fixdt(1, 16)  OutScaling=2^0  SampleTime=dt
  Select Homing Joint : Gain  Gain=diag([1;1;1;1;1;1;1;0;0])  Multiplication=Matrix(K*u)  ParameterDataType=fixdt(1, 16)  ParameterScaling=2^0  OutDataType=fixdt(1, 16)  OutScaling=2^0  SampleTime=dt
  Sum : Sum  Inputs=|+-  OutDataType=fixdt(1, 16)  OutScaling=2^0  SampleTime=dt
  Sum1 : Sum  Inputs=|++  OutDataType=fixdt(1, 16)  OutScaling=2^0
  Terminator : Terminator
  Terminator1 : Terminator
  Unit Delay : UnitDelay  X0=zeros(9,1)  SampleTime=-1
  Unit Delay1 : UnitDelay  X0=false(9,1)  SampleTime=-1
  dt : Constant  Value=dt  OutDataType=fixdt(1, 16)  OutScaling=2^0  SampleTime=dt
  home voltage : Constant  Value=right_arm_home_voltage  OutDataType=fixdt(1, 16)  OutScaling=2^0  SampleTime=dt
  q des : Outport  OutDataType=fixdt(1, 16)  OutScaling=2^0  InitialOutput=zeros(9,1)
  wires:
  sensors/1 -> Bus Selector/1
  Sum/1 -> Select Homing Joint/1
  home voltage/1 -> Sum/1
  Bus Selector/1 -> Demux/1  "<right arm pots>"
  Demux/1 -> Sum/2
  Demux/2 -> Terminator/1
  Homing Completion/1(Homed) -> Terminator1/1
  Select Homing Joint/1 -> Homing Direction/1
  HomingRoughVelocity/1 -> Fine_Rough_Homing_Switch/4(HomingVel)
  Unit Delay1/1 -> Fine_Rough_Homing_Switch/6(PrevHomedJoint)
  Fine_Rough_Homing_Switch/3(HomedJoint) -> Unit Delay1/1
  HomingRoughEps/1 -> Fine_Rough_Homing_Switch/3(ERROR_eps)
  dt/1 -> Fine_Rough_Homing_Switch/2(dt)
  Unit Delay/1 -> Fine_Rough_Homing_Switch/5(q_cur)
  Fine_Rough_Homing_Switch/2(q_des) -> Unit Delay/1, Sum1/2
  Fine_Rough_Homing_Switch/1(EnableFineHoming) -> Fine Homing - Integral Control/Enable
  Fine Homing - Integral Control/1(q_des_fine) -> Sum1/1
  Sum1/1 -> q des/1
  Homing Direction/1 -> Homing Completion/1(u), Fine_Rough_Homing_Switch/1(error), Fine Homing - Integral Control/1(error)
  HomingFineEps/1 -> Homing Completion/2(EPS)

== system irep_single_axis/Trajectory Planner/Left Arm/Low Level/Home Procedure2 ==
  note: Before the Gains for Jonit 8 and Joint 9 were [-1 -1].
      | Temporarily we disable the homing for those two joints, the values now are [0 0]
  sensors : Inport  OutDataType=fixdt(1, 16)  OutScaling=2^0
  Enable : EnablePort
  Bus Selector : BusSelector  OutputSignals=A/D signals.left arm pots
  Demux : Demux  Outputs=[9 1]
  Discrete-Time Integrator : DiscreteIntegrator  SampleTime=dt  OutDataType=fixdt(1, 16)  OutScaling=2^0  LimitOutput=on  UpperSaturationLimit=8  LowerSaturationLimit=-8  ICPrevOutput=DiscIntNeverNeededParam  ICPrevScaledInput=DiscIntNeverNeededParam
  Gain : Gain  Gain=diag([-1;-1;-1;1;1;-1;-1;1;-1])*0.5  Multiplication=Matrix(K*u)  ParameterDataType=fixdt(1, 16)  ParameterScaling=2^0  OutDataType=fixdt(1, 16)  OutScaling=2^0  SampleTime=dt
  Homing Completion : Stateflow chart  TreatAsAtomicUnit=on
  Sum : Sum  Inputs=|+-  OutDataType=fixdt(1, 16)  OutScaling=2^0  SampleTime=dt
  Terminator : Terminator
  Terminator1 : Terminator
  home voltage : Constant  Value=left_arm_home_voltage  OutDataType=fixdt(1, 16)  OutScaling=2^0  SampleTime=dt
  q des : Outport  OutDataType=fixdt(1, 16)  OutScaling=2^0  InitialOutput=zeros(9,1)
  wires:
  Homing Completion/1(y) -> Terminator1/1
  Demux/2 -> Terminator/1
  Demux/1 -> Sum/2
  Bus Selector/1 -> Demux/1  "<left arm pots>"
  Discrete-Time Integrator/1 -> q des/1
  Gain/1 -> Discrete-Time Integrator/1
  home voltage/1 -> Sum/1
  Sum/1 -> Homing Completion/1(u), Gain/1
  sensors/1 -> Bus Selector/1

== system irep_single_axis/Trajectory Planner/Left Arm/Low Level/Joint Space ==
  Enable : EnablePort
  q desired : Constant  Value=zeros(9,1)  OutDataType=fixdt(1, 16)  OutScaling=2^0  SampleTime=dt
  q des : Outport  OutDataType=fixdt(1, 16)  OutScaling=2^0
  wires:
  q desired/1 -> q des/1

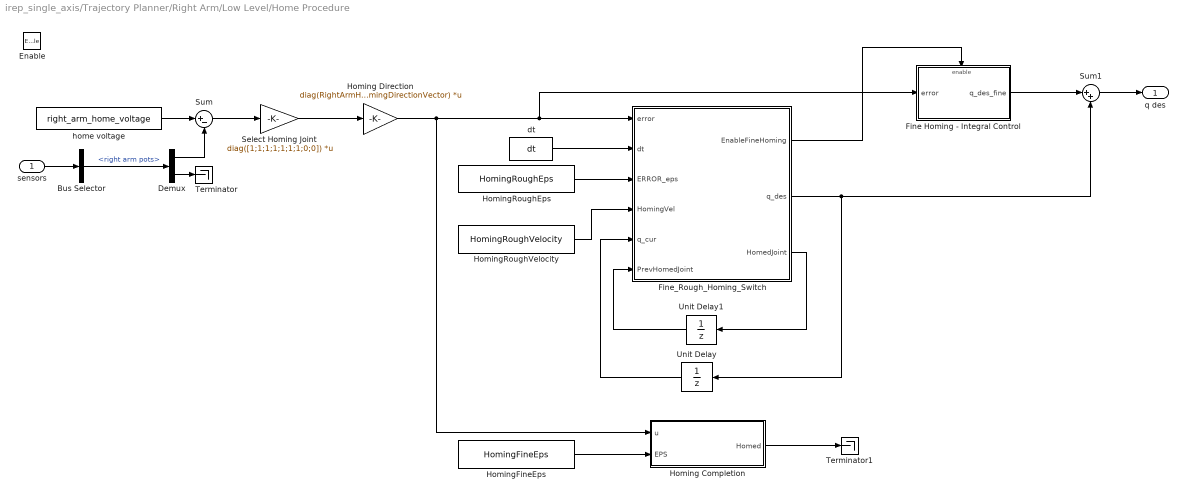
== system irep_single_axis/Trajectory Planner/Right Arm/Low Level/Home Procedure ==
  sensors : Inport  OutDataType=fixdt(1, 16)  OutScaling=2^0
  Enable : EnablePort
  Bus Selector : BusSelector  OutputSignals=A/D signals.right arm pots
  Demux : Demux  Outputs=[9 1]
  Fine Homing - Integral Control : Subsystem
  Fine_Rough_Homing_Switch : Stateflow chart  TreatAsAtomicUnit=on
  Homing Completion : Stateflow chart  TreatAsAtomicUnit=on
  Homing Direction : Gain  Gain=diag(RightArmHomingDirectionVector)  Multiplication=Matrix(K*u)  ParameterDataType=fixdt(1, 16)  ParameterScaling=2^0  OutDataType=fixdt(1, 16)  OutScaling=2^0  SampleTime=dt
  HomingFineEps : Constant  Value=HomingFineEps  OutDataType=fixdt(1, 16)  OutScaling=2^0  SampleTime=dt
  HomingRoughEps : Constant  Value=HomingRoughEps  OutDataType=fixdt(1, 16)  OutScaling=2^0  SampleTime=dt
  HomingRoughVelocity : Constant  Value=HomingRoughVelocity  OutDataType=fixdt(1, 16)  OutScaling=2^0  SampleTime=dt
  Select Homing Joint : Gain  Gain=diag([1;1;1;1;1;1;1;0;0])  Multiplication=Matrix(K*u)  ParameterDataType=fixdt(1, 16)  ParameterScaling=2^0  OutDataType=fixdt(1, 16)  OutScaling=2^0  SampleTime=dt
  Sum : Sum  Inputs=|+-  OutDataType=fixdt(1, 16)  OutScaling=2^0  SampleTime=dt
  Sum1 : Sum  Inputs=|++  OutDataType=fixdt(1, 16)  OutScaling=2^0
  Terminator : Terminator
  Terminator1 : Terminator
  Unit Delay : UnitDelay  X0=zeros(9,1)  SampleTime=-1
  Unit Delay1 : UnitDelay  X0=false(9,1)  SampleTime=-1
  dt : Constant  Value=dt  OutDataType=fixdt(1, 16)  OutScaling=2^0  SampleTime=dt
  home voltage : Constant  Value=right_arm_home_voltage  OutDataType=fixdt(1, 16)  OutScaling=2^0  SampleTime=dt
  q des : Outport  OutDataType=fixdt(1, 16)  OutScaling=2^0  InitialOutput=zeros(9,1)
  wires:
  sensors/1 -> Bus Selector/1
  Sum/1 -> Select Homing Joint/1
  home voltage/1 -> Sum/1
  Bus Selector/1 -> Demux/1  "<right arm pots>"
  Demux/1 -> Sum/2
  Demux/2 -> Terminator/1
  Homing Completion/1(Homed) -> Terminator1/1
  Select Homing Joint/1 -> Homing Direction/1
  HomingRoughVelocity/1 -> Fine_Rough_Homing_Switch/4(HomingVel)
  Unit Delay1/1 -> Fine_Rough_Homing_Switch/6(PrevHomedJoint)
  Fine_Rough_Homing_Switch/3(HomedJoint) -> Unit Delay1/1
  HomingRoughEps/1 -> Fine_Rough_Homing_Switch/3(ERROR_eps)
  dt/1 -> Fine_Rough_Homing_Switch/2(dt)
  Unit Delay/1 -> Fine_Rough_Homing_Switch/5(q_cur)
  Fine_Rough_Homing_Switch/2(q_des) -> Unit Delay/1, Sum1/2
  Fine_Rough_Homing_Switch/1(EnableFineHoming) -> Fine Homing - Integral Control/Enable
  Fine Homing - Integral Control/1(q_des_fine) -> Sum1/1
  Sum1/1 -> q des/1
  Homing Direction/1 -> Homing Completion/1(u), Fine_Rough_Homing_Switch/1(error), Fine Homing - Integral Control/1(error)
  HomingFineEps/1 -> Homing Completion/2(EPS)

== system irep_single_axis/Trajectory Planner/Right Arm/Low Level/Joint Space ==
  Enable : EnablePort
  q desired : Constant  Value=zeros(9,1)  OutDataType=fixdt(1, 16)  OutScaling=2^0  SampleTime=dt
  q des : Outport  OutDataType=fixdt(1, 16)  OutScaling=2^0
  wires:
  q desired/1 -> q des/1

== system irep_single_axis/In-Vivo System/ATI FT Sensor/ATI Force Torque Sensor/Enabled Subsystem1/Voltage Filter Bias ==
  V_in : Inport
  Discrete FIR Filter : DiscreteFir  CoefSource=Input port
  Gain : Gain  Gain=1/N_ATI_bias
  filter_coeffs : Constant  Value=filter_coeffs_ATI_bias
  V_Out : Outport
  wires:
  Gain/1 -> V_Out/1
  filter_coeffs/1 -> Discrete FIR Filter/2
  Discrete FIR Filter/1 -> Gain/1
  V_in/1 -> Discrete FIR Filter/1

== system irep_single_axis/Trajectory Planner/Left Arm/Low Level/Home Procedure/Fine Homing - Integral Control ==
  error : Inport
  Enable : EnablePort  StatesWhenEnabling=reset
  Discrete-Time Integrator : DiscreteIntegrator  SampleTime=dt  OutDataType=fixdt(1, 16)  OutScaling=2^0  LimitOutput=on  UpperSaturationLimit=8  LowerSaturationLimit=-8  ICPrevOutput=DiscIntNeverNeededParam  ICPrevScaledInput=DiscIntNeverNeededParam
  Integral Gain : Gain  Gain=diag(RightArmHomingIntGain)  Multiplication=Matrix(K*u)  ParameterDataType=fixdt(1, 16)  ParameterScaling=2^0  OutDataType=fixdt(1, 16)  OutScaling=2^0  SampleTime=dt
  q_des_fine : Outport  InitialOutput=zeros(9,1)
  wires:
  error/1 -> Integral Gain/1
  Discrete-Time Integrator/1 -> q_des_fine/1
  Integral Gain/1 -> Discrete-Time Integrator/1

== system irep_single_axis/Trajectory Planner/Right Arm/Low Level/Home Procedure/Fine Homing - Integral Control ==
  error : Inport
  Enable : EnablePort  StatesWhenEnabling=reset
  Discrete-Time Integrator : DiscreteIntegrator  SampleTime=dt  OutDataType=fixdt(1, 16)  OutScaling=2^0  LimitOutput=on  UpperSaturationLimit=8  LowerSaturationLimit=-8  ICPrevOutput=DiscIntNeverNeededParam  ICPrevScaledInput=DiscIntNeverNeededParam
  Integral Gain : Gain  Gain=diag(RightArmHomingIntGain)  Multiplication=Matrix(K*u)  ParameterDataType=fixdt(1, 16)  ParameterScaling=2^0  OutDataType=fixdt(1, 16)  OutScaling=2^0  SampleTime=dt
  q_des_fine : Outport  InitialOutput=zeros(9,1)
  wires:
  error/1 -> Integral Gain/1
  Discrete-Time Integrator/1 -> q_des_fine/1
  Integral Gain/1 -> Discrete-Time Integrator/1

== matlab function Trajectory Planner/Camera/Joint Space/5th Order Polynomial/Embedded MATLAB Function ==
  data: p output double; p_des input double; p_curr input double; tf input double; tc input double; pdot output double; pdotdot output double; conf input double; confn output double; t0 input double; t0n output double; p0n output double; p0 input double; enable input double; RECORD output double
function [p,pdot,pdotdot,confn,t0n,p0n,RECORD] = fifth_order_p(p_des,p_curr,tf,tc,conf,t0,p0,enable)

n = 3;
RECORD = 0;

if enable == 0                  % Configuration space is not used (pdot = 0). 
    p = p_curr;
    pdotdot = zeros(n,1);
    pdot = zeros(n,1);          % However we do want to record the current 
    confn = 0;                  % position in order to be ready as soon 
    t0n = tc;                   % as the enable becomes 1. 
    p0n = p_curr;
else
    if (p_des-p0)'*(p_des-p0) > 0
        if conf == 0                % conf = 0 means that the 5th order poly 
            p0n = p0;               % is not configured for the desired trajectory.
            t0n = tc;               % Therefore, the block is initialized.
            confn = 1;
            pdot = zeros(n,1);
            p = p0;
            pdotdot = zeros(n,1);
        else
            p0n = p0;
            t0n = t0;
            confn = conf;
            % 5th order polynomial
            a0 = p0;
            a4 = -15*(p_des-p0);
            a3 = -2/3 * a4;
            a5 = -2/5 * a4;
            t = tc-t0;
            tau = t/tf;
            if t < tf
                RECORD = 1;
                p = a0 + a3 * tau^3 + a4 * tau^4 + a5 * tau^5;
                pdot = 3*a3*t^2/tf^3 + 4*a4*t^3/tf^4 + 5*a5*t^4/tf^5;
                pdotdot = 6*a3*t/tf^3 + 12*a4*t^2/tf^4 + 20*a5*t^3/tf^5;
            else
                p = p_des;
                pdot = zeros(n,1);
                pdotdot = zeros(n,1);
                p0n = p_des;
            end
        end
    else
        p = p_des;
        pdot = zeros(n,1);
        pdotdot = zeros(n,1);
        confn = 0;
        p0n = p0;
        t0n = t0;
    end
end
%------------------------------------------------------------------------

== matlab function Trajectory Planner/Camera/Contact Detection/Embedded MATLAB Function ==
  data: F input double; c output double; thresh input double
function c= fcn(F,thresh)
%#eml
if norm(F)>thresh
    c = 1;
else
    c = 0;
end

== matlab function Trajectory Planner/Camera/Joint Space/fine  motion/Embedded MATLAB Function ==
  data: p_des output double; enable input double; go input double; dt input double; velocity input double; p0 input double; p_cur input double
function p_des = fcn(enable,go,dt,velocity,p0,p_cur)
%#eml
if enable
    if go
        p_des = p_cur + dt*velocity;
    else
        p_des = p_cur;
    end
else
    p_des = p0;
end

== matlab function Trajectory Planner/Camera/Joint Space/Embedded MATLAB Function ==
  data: F input double; go output double; thresh input double
function go= fcn(F,thresh)
%#eml
if norm(F)>thresh
    go = 0;
else
    go = 1;
end

== matlab function Trajectory Planner/Camera/Joint Space/Sine Motion/Embedded MATLAB Function ==
  data: p_des output double; p0n output double; go input double; tc input double; freq input double; amp input double; p_cur input double; p0 input double; t0 input double; t0n output double
function [p_des,p0n,t0n] = fcn(go,tc,freq,amp,p_cur,p0,t0)
%#eml
if go
    t = tc - t0;
    p_des = p0 + amp*sin(2*pi*freq*t)*ones(3,1);
    t0n = t0;
    p0n = p0;
else
    p_des = p_cur;
    p0n = p_cur;
    t0n = tc;
end

== matlab function In-Vivo System/ATI FT Sensor/ATI Force Torque Sensor/Convert from Voltage to Wrench  ==
  data: V input double; W output double; A input double; inv_T input double
function W = Convert_Function(V,A,inv_T)%A_vec,p)

W = inv_T*A*V;

== matlab function In-Vivo System/ATI FT Sensor/ATI Force Torque Sensor/FT Flag func ==
  data: clock input double; flag output double
function flag = fcn(clock)
%#eml
if clock<=6
    flag=1;
else
    flag=0;
end

== matlab function Trajectory Planner/Right Arm/Low Level/Home Procedure/Homing Completion ==
  data: u input double; Homed output double; EPS input double
function Homed = fcn(u,EPS)
%#eml
u = abs(u);
Homed = (u<=EPS);

== matlab function Trajectory Planner/Left Arm/Low Level/Not And ==
  data: connected input double; enable output double; enable_home input double
function enable = fcn(connected,enable_home)
%#eml
FB = connected(1,1); % FB for front pot board
RB = connected(2,1); % RB for Rear pot board
% FB=0 means that the potentiometer cable is connected.
% to ensure both connceted, FB+RB=0.
if (FB+RB) == 0 && enable_home == 1
    enable = 1;
else
    enable = 0;
end

== matlab function Trajectory Planner/Right Arm/Low Level/Not And ==
  data: connected input double; enable output double; enable_home input double
%This block ensures that the potentiometer cables are connected before 
% homing can proceed
function enable = fcn(connected,enable_home)
%#eml
FB = connected(1,1); % FB for front pot board
RB = connected(2,1); % RB for Rear pot board
% FB=0 means that the potentiometer cable is connected.
% to ensure both connceted, FB+RB=0.
if (FB+RB) == 0 && enable_home == 1
    enable = 1;
else
    enable = 0;
end

== matlab function In-Vivo System/Potentiometers/Initialize Joystick/Embedded MATLAB Function ==
  data: V output double; u_curr input double; v_zero output double; t input double; u_prev input double
function [V,v_zero] = fcn(u_curr,t,u_prev)
%#eml

if t == 2 
    V = u_curr;
    v_zero = u_curr;
else
    V = u_curr - u_prev;
    v_zero = u_prev;
end

== matlab function Trajectory Planner/Right Arm/Low Level/Home Procedure/Fine_Rough_Homing_Switch ==
  data: EnableFineHoming output double; error input double; dt input double; q_des output double; ERROR_eps input double; HomingVel input double; q_cur input double; HomedJoint output boolean; PrevHomedJoint input boolean
function [EnableFineHoming,q_des,HomedJoint] = fcn(error, dt,ERROR_eps,HomingVel,q_cur,PrevHomedJoint)
%#eml
%   By Long Wang, 2015/1/20
%   Input:
%       error       -> the current error in potentiometers
%       ERROR_eps   -> the tolenrace defined in potentiometers which will determine if within rough control range 
%       q_cur       -> the previous command
%       PrevHomedJoint  -> if homed detected from the previous time step
%       HomingVel       -> the joint velocity to command if the joint is rough homing mode
HomedJoint = (abs(error)<ERROR_eps);
HomedJoint = (HomedJoint|PrevHomedJoint); 
%   if the joint was detected homed previously, it will be forever seen as homed
%   to avoid noise on pots.
if sum(HomedJoint)==9
    % all joints are in rough homing control range, need to use fine homing
    q_des = q_cur; % stays the previous command
    EnableFineHoming = 1;
else
    %   not all joints are in rough homing control range
    %   the ones which are not, need to give constant velocity command
    %   And the other joints will be waiting untill all the joints are in Fine Homing mode
    EnableFineHoming = 0;
    velocity = (1-HomedJoint).*sign(error).*HomingVel; 
    q_des = q_cur + velocity*dt;
end
